simulink model "Noa_Nofusion_angle"  (R2020b)
settings: Solver=FixedStepDiscrete  StartTime=0.0  StopTime=Inf  FixedStep=0.01  RelTol=1e-3
PostLoadFcn:
  | if any(exist('dsrtsu_mdlpostloadfcn', 'file') ~= 0), dsrtsu_mdlpostloadfcn('Execute', bdroot); end
InitFcn:
  | , if any(exist('rtifpga_mdlclblib', 'file') ~= 0), rtifpga_mdlclblib('Init', bdroot); end,
  | , if any(exist('dsmpb_private', 'file') ~= 0), dsmpb_private('dsmpb_mdlclblib', 'Init', bdroot); end,
undefined symbols (not defined in the file): ACC_TimeGap_DecSetSwt, ACC_TimeGap_IncSetSwt, AccelPedalPosn, AccelPedalPosnVldty, AccelPedlPosnDiagc, AccPedalOverride, ACU_ShiftInProgress, ADAS_Posn_CurLane, AESSwtReq, ALC_SwtReq, BrkPedalSts, CC_ACC_CANCEL_OFFSwt, CC_ACC_CRUISE_OFFSwt, CC_ACC_DecSetSpd_SetSwt, CC_ACC_IncSetSpd_ResuSwt, CC_ACCSwtErr, CharSpd_ms, CSA_NODE, CURRENT_GEAR, CurrentGearValid, DiscIntNeverNeededParam, DrvDoorSts, DrvSBR, DrvTrqReqOvld, ECMACCInterface, ECMRespACC, ELKSwtReq, EngLimpHomeSts, EngSpd, EngState, EngState_PHEV, EngTrqMaxActSpd, EngTrqMinAct, EPS_DrvInpTrqVal_HighReslolution, EPS_FailSts, EPS_LKATorqOvrlDlvd, EPS_LKATorqOvrlDlvdVld, EPS_LKATrqOvlDlvdSts, EPS_SteerMod, EPS_TrqSnsrSts, EQ4_APPINFO, EQ4_LA_ELEM, EQ4_LA_HDR, EQ4_LAP_ELEM, EQ4_LAP_HDR, EQ4_LH_ELEM, EQ4_LH_HDR, EQ4_LRE_ELEM, EQ4_LRE_HDR, ESS_PedSwtReq, ESS_VehSwtReq, FFogLmpSts_F_Pbox, FLWheelDriveDirection, FLWheelSpd, FrntWiprSwtSts, FrntWshrSwtSts, FRWheelDriveDirection, FRWheelSpd, HazardLmpSwtSts, HCU_AccelPedalPosn_Diag ... (+151)
libraries: simulink x138, dsmpblib x33, canfdmsglib x10
(part 16 of 17)

== matlab function Noa_Nofusion_angle/CR_RSDS_Input/CR_R_Bus/CR ==
  data: RadarID input uint8 size=1; ID input uint8 size=6; Dx input single size=6; Dy input single size=6; Vx input single size=6; Vy input single size=6; Ax input single size=6; ObjIDK1 input uint8 size=6; P output uint8 size=6; ObjDx output single size=6; ObjDy output single size=6; ObjVx output single size=6; ObjVy output single size=6; ObjAx output single size=6; ObjMoveSts output uint8 size=6; ObjFusType output uint8 size=6; ObjID output uint8 size=6; ObjAgeK1 input uint8 size=6; ObjAge output uint8 size=6
function [P,ObjDx,ObjDy,ObjVx,ObjVy,ObjAx,ObjMoveSts,ObjFusType,ObjID,ObjAge] =...
    DataT(RadarID,ID,Dx,Dy,Vx,Vy,Ax,ObjIDK1,ObjAgeK1)

if RadarID==uint8(1)
    FusFac = 4;
elseif RadarID==uint8(2)
    FusFac = 8;
elseif RadarID==uint8(3)
    FusFac = 16;
else
    FusFac = 32;
end

ObjID = uint8(zeros(6,1));
ObjDx = single(zeros(6,1));
ObjDy = single(zeros(6,1));
ObjVx = single(zeros(6,1));
ObjVy = single(zeros(6,1));
ObjAx = single(zeros(6,1));
ObjAge = uint8(ones(6,1));
ObjMoveSts = uint8(2*ones(6,1));
ObjFusType = uint8(FusFac*ones(6,1));

T = uint8(zeros(6,1));
P = uint8(zeros(6,1));
Index01 = uint8(zeros(6,1));
Index02 = uint8(zeros(6,1));
M = uint8(0);
N = uint8(0);
w = uint8(0);

for i=uint8(1):uint8(6)
    for j=uint8(1):uint8(6)
        if ID(i)==ObjIDK1(j) && ID(i)>uint8(0)
            T(j) = i;
            P(i) = j;
        end
    end
end

for j=uint8(1):uint8(6)
    if T(j)==uint8(0)
        if ObjIDK1(j)==uint8(0)
            N = N + uint8(1);
            Index01(N) = j;
        else
            M = M + uint8(1);
            Index02(M) = j;
        end
    end
end

for i=uint8(1):uint8(6)
    if P(i)==uint8(0) && ID(i)>uint8(0)
        w = w + uint8(1);
        if w<=N
            P(i) = Index01(w);
        else
            P(i) = Index02(w - N);
        end
    elseif P(i)>uint8(0)
        ObjAge(P(i)) = min(ObjAgeK1(i) + uint8(1),uint8(255));
    end
    if P(i)>uint8(0)
       ObjID(P(i)) = ID(i);
       ObjDx(P(i)) = Dx(i);
       ObjDy(P(i)) = Dy(i);
       ObjVx(P(i)) = Vx(i);
       ObjVy(P(i)) = Vy(i);
       ObjAx(P(i)) = Ax(i);
    end
end
for i=uint8(1):uint8(6)
    if ObjID(i)==uint8(0)
        ObjAge(i) = uint8(0);
        ObjMoveSts(i) = uint8(0);
        ObjFusType(i) = uint8(0);
    end
end
end

== matlab function Noa_Nofusion_angle/TOS/Subsystem1/ACCOSM/HWA_Task100ms1/OTL1/MATLAB Function ==
  data: t input single; Valid output boolean; CutIn_b input boolean; ValidK1 input boolean
function Valid = fcn(t,CutIn_b,ValidK1)

if t<0.1
    Valid = false;
else
    if CutIn_b==false
       Valid = true; 
    else
       Valid = ValidK1;
    end
end

== matlab function Noa_Nofusion_angle/CR_RSDS_Input/MATLAB Function1 ==
  data: ObjNumber input uint8 size=1; ObjPrio output single size=24; ObjID input uint8 size=24; ObjDx input single size=24; ObjMatrix output single size=24
function [ObjPrio,ObjMatrix] = fcn(ObjNumber,ObjID,ObjDx)
%#codegen
ObjPrio = single(zeros(24,1));

for i=1:ObjNumber
    if ObjID(i)>0
        ObjPrio(i)=single(255) - abs(ObjDx(i));
    else
        ObjPrio(i)=single(0);
    end
end

ObjMatrix=ObjPrio;

t_h=1;
while 1
    t_h = t_h*3+1;
    if t_h>=ObjNumber
        break;
    end
end

%   t_h = 121;
while 1
    t_h = fix(t_h/3);
    for i=(t_h+1):ObjNumber
        j=i;
        t_zw=ObjMatrix(i);
        while (j>t_h)&&(t_zw<ObjMatrix(j-t_h))
            ObjMatrix(j)=ObjMatrix(j-t_h);
            j=j-t_h;
        end
        ObjMatrix(j)=t_zw;
    end
    if t_h==1
        break;
    end
end
end

== matlab function Noa_Nofusion_angle/CR_RSDS_Input/MATLAB Function2 ==
  data: Prio input single size=24; Matrix input single size=24; ID input uint8 size=24; ObjID output uint8 size=11; Dx input single size=24; Dy input single size=24; ObjDx output single size=11; Vx input single size=24; Vy input single size=24; Ax input single size=24; Age input uint8 size=24; MoveSts input uint8 size=24; ObjDy output single size=11; ObjVx output single size=11; ObjVy output single size=11; ObjAx output single size=11; ObjAge output uint8 size=11; ObjMoveSts output uint8 size=11; FusType input uint8 size=24; ObjFusType output uint8 size=11
function [ObjID,ObjDx,ObjDy,ObjVx,ObjVy,ObjAx,ObjAge,ObjMoveSts,ObjFusType] =...
    fcn(Prio,Matrix,ID,Dx,Dy,Vx,Vy,Ax,Age,MoveSts,FusType)
%#codegen
ObjPrioLimit = Matrix(24-11);
ObjID = uint8(zeros(11,1));
ObjDx = single(zeros(11,1));
ObjDy = single(zeros(11,1));
ObjVx = single(zeros(11,1));
ObjVy = single(zeros(11,1));
ObjAx = single(zeros(11,1));
ObjAge = uint8(zeros(11,1));
ObjMoveSts = uint8(zeros(11,1));
ObjFusType = uint8(zeros(11,1));
Num = uint8(0);

for i=1:24
  if ID(i)>0 && Prio(i)>ObjPrioLimit
      Num = Num + uint8(1);
      ObjID(Num) = uint8(i);
      ObjDx(Num) = Dx(i);
      ObjDy(Num) = Dy(i);
      ObjVx(Num) = Vx(i);
      ObjVy(Num) = Vy(i);
      ObjAx(Num) = Ax(i);
      ObjAge(Num) = Age(i);
      ObjMoveSts(Num) = MoveSts(i);
      ObjFusType(Num) = FusType(i);
  end
end

== matlab function Noa_Nofusion_angle/CR_RSDS_Input/RSDS_L_Bus/RSDS_L ==
  data: RadarID input uint8 size=1; ID input uint8 size=6; Dx input single size=6; Dy input single size=6; Vx input single size=6; Vy input single size=6; Ax input single size=6; ObjIDK1 input uint8 size=6; P output uint8 size=6; ObjDx output single size=6; ObjDy output single size=6; ObjVx output single size=6; ObjVy output single size=6; ObjAx output single size=6; ObjMoveSts output uint8 size=6; ObjFusType output uint8 size=6; ObjID output uint8 size=6; ObjAgeK1 input uint8 size=6; ObjAge output uint8 size=6
function [P,ObjDx,ObjDy,ObjVx,ObjVy,ObjAx,ObjMoveSts,ObjFusType,ObjID,ObjAge] =...
    DataT(RadarID,ID,Dx,Dy,Vx,Vy,Ax,ObjIDK1,ObjAgeK1)

if RadarID==uint8(1)
    FusFac = 4;
elseif RadarID==uint8(2)
    FusFac = 8;
elseif RadarID==uint8(3)
    FusFac = 16;
else
    FusFac = 32;
end

ObjID = uint8(zeros(6,1));
ObjDx = single(zeros(6,1));
ObjDy = single(zeros(6,1));
ObjVx = single(zeros(6,1));
ObjVy = single(zeros(6,1));
ObjAx = single(zeros(6,1));
ObjAge = uint8(ones(6,1));
ObjMoveSts = uint8(2*ones(6,1));
ObjFusType = uint8(FusFac*ones(6,1));

T = uint8(zeros(6,1));
P = uint8(zeros(6,1));
Index01 = uint8(zeros(6,1));
Index02 = uint8(zeros(6,1));
M = uint8(0);
N = uint8(0);
w = uint8(0);

for i=uint8(1):uint8(6)
    for j=uint8(1):uint8(6)
        if ID(i)==ObjIDK1(j) && ID(i)>uint8(0)
            T(j) = i;
            P(i) = j;
        end
    end
end

for j=uint8(1):uint8(6)
    if T(j)==uint8(0)
        if ObjIDK1(j)==uint8(0)
            N = N + uint8(1);
            Index01(N) = j;
        else
            M = M + uint8(1);
            Index02(M) = j;
        end
    end
end

for i=uint8(1):uint8(6)
    if P(i)==uint8(0) && ID(i)>uint8(0)
        w = w + uint8(1);
        if w<=N
            P(i) = Index01(w);
        else
            P(i) = Index02(w - N);
        end
    elseif P(i)>uint8(0)
        ObjAge(P(i)) = min(ObjAgeK1(i) + uint8(1),uint8(255));
    end
    if P(i)>uint8(0)
       ObjID(P(i)) = ID(i);
       ObjDx(P(i)) = Dx(i);
       ObjDy(P(i)) = Dy(i);
       ObjVx(P(i)) = Vx(i);
       ObjVy(P(i)) = Vy(i);
       ObjAx(P(i)) = Ax(i);
    end
end
for i=uint8(1):uint8(6)
    if ObjID(i)==uint8(0)
        ObjAge(i) = uint8(0);
        ObjMoveSts(i) = uint8(0);
        ObjFusType(i) = uint8(0);
    end
end
end

== matlab function Noa_Nofusion_angle/CR_RSDS_Input/RSDS_R_Bus/RSDS_R ==
  data: RadarID input uint8 size=1; ID input uint8 size=6; Dx input single size=6; Dy input single size=6; Vx input single size=6; Vy input single size=6; Ax input single size=6; ObjIDK1 input uint8 size=6; P output uint8 size=6; ObjDx output single size=6; ObjDy output single size=6; ObjVx output single size=6; ObjVy output single size=6; ObjAx output single size=6; ObjMoveSts output uint8 size=6; ObjFusType output uint8 size=6; ObjID output uint8 size=6; ObjAgeK1 input uint8 size=6; ObjAge output uint8 size=6
function [P,ObjDx,ObjDy,ObjVx,ObjVy,ObjAx,ObjMoveSts,ObjFusType,ObjID,ObjAge] =...
    DataT(RadarID,ID,Dx,Dy,Vx,Vy,Ax,ObjIDK1,ObjAgeK1)

if RadarID==uint8(1)
    FusFac = 4;
elseif RadarID==uint8(2)
    FusFac = 8;
elseif RadarID==uint8(3)
    FusFac = 16;
else
    FusFac = 32;
end

ObjID = uint8(zeros(6,1));
ObjDx = single(zeros(6,1));
ObjDy = single(zeros(6,1));
ObjVx = single(zeros(6,1));
ObjVy = single(zeros(6,1));
ObjAx = single(zeros(6,1));
ObjAge = uint8(ones(6,1));
ObjMoveSts = uint8(2*ones(6,1));
ObjFusType = uint8(FusFac*ones(6,1));

T = uint8(zeros(6,1));
P = uint8(zeros(6,1));
Index01 = uint8(zeros(6,1));
Index02 = uint8(zeros(6,1));
M = uint8(0);
N = uint8(0);
w = uint8(0);

for i=uint8(1):uint8(6)
    for j=uint8(1):uint8(6)
        if ID(i)==ObjIDK1(j) && ID(i)>uint8(0)
            T(j) = i;
            P(i) = j;
        end
    end
end

for j=uint8(1):uint8(6)
    if T(j)==uint8(0)
        if ObjIDK1(j)==uint8(0)
            N = N + uint8(1);
            Index01(N) = j;
        else
            M = M + uint8(1);
            Index02(M) = j;
        end
    end
end

for i=uint8(1):uint8(6)
    if P(i)==uint8(0) && ID(i)>uint8(0)
        w = w + uint8(1);
        if w<=N
            P(i) = Index01(w);
        else
            P(i) = Index02(w - N);
        end
    elseif P(i)>uint8(0)
        ObjAge(P(i)) = min(ObjAgeK1(i) + uint8(1),uint8(255));
    end
    if P(i)>uint8(0)
       ObjID(P(i)) = ID(i);
       ObjDx(P(i)) = Dx(i);
       ObjDy(P(i)) = Dy(i);
       ObjVx(P(i)) = Vx(i);
       ObjVy(P(i)) = Vy(i);
       ObjAx(P(i)) = Ax(i);
    end
end
for i=uint8(1):uint8(6)
    if ObjID(i)==uint8(0)
        ObjAge(i) = uint8(0);
        ObjMoveSts(i) = uint8(0);
        ObjFusType(i) = uint8(0);
    end
end
end

== matlab function Noa_Nofusion_angle/TOS/Subsystem1/ACCOSM/HWA_Task100ms1/OTL1/P0TrajHistCalc01 ==
  data: P0Dyc output; vRef input; tCycle input single; tSameHandle input single; CutIn input; P0Dx input single; P0Dy input single; P0TrajHistNum output uint8; EgoDDeltaX input single; EgoDDeltaY input single; EgoCosOfPsi input single; EgoSinOfPsi input single; TarLineValid input; TarLineA2 input; TarLineA1 input; TarLineA0 input; P0TrajHistDxv output single; P0TrajHistDyv output single; P0TrajHistNumK1 input uint8; P0TrajHistDxvK1 input single; P0TrajHistDyvK1 input single
function [P0Dyc,P0TrajHistNum,P0TrajHistDxv,P0TrajHistDyv]...
    = fcn(vRef, tCycle,tSameHandle,CutIn, P0Dx,P0Dy,EgoDDeltaX,EgoDDeltaY,EgoCosOfPsi,EgoSinOfPsi,...
    TarLineValid,TarLineA2,TarLineA1,TarLineA0,...
    P0TrajHistNumK1,P0TrajHistDxvK1,P0TrajHistDyvK1)
%#codegen
P0TrajHistNum = P0TrajHistNumK1;
P0TrajHistDxv = P0TrajHistDxvK1;
P0TrajHistDyv = P0TrajHistDyvK1;

if TarLineValid
    temp1 = TarLineA2*P0Dx*P0Dx + TarLineA1*P0Dx + TarLineA0;
    P0Dyc = P0Dy - temp1;
else
    P0Dyc = single(255);
end
                
if tSameHandle==0
    P0TrajHistNum = uint8(0);
    P0TrajHistDxv = single(zeros(24,1));
    P0TrajHistDyv = single(zeros(24,1));
else
    if tSameHandle==tCycle
        if (CutIn&&abs(P0Dyc)>0.5) || (abs(P0Dyc)>0.8)||(vRef>8)
            P0TrajHistDxv(1) = P0Dx;
            P0TrajHistDyv(1) = P0Dy;
            P0TrajHistNum = uint8(1);
        else
            P0TrajHistDxv(1) = P0Dx;
            P0TrajHistDyv(1) = P0Dy;
            P0TrajHistNum = uint8(1);
            
            if TarLineValid
                P0TrajHistDxv(2) = 0.6*P0Dx;
                temp2 = 0.36*TarLineA2*P0Dx*P0Dx + 0.6*TarLineA1*P0Dx + TarLineA0;
                P0TrajHistDyv(2) = P0Dyc + temp2;
                
                P0TrajHistDxv(3) = 0.3*P0Dx;
                temp3 = 0.09*TarLineA2*P0Dx*P0Dx + 0.3*TarLineA1*P0Dx + TarLineA0;
                P0TrajHistDyv(3) = P0Dyc + temp3;
                
                P0TrajHistDxv(4) = single(-1);
                temp4 = TarLineA2 - TarLineA1 + TarLineA0;
                P0TrajHistDyv(4) = P0Dyc + temp4;
                
                P0TrajHistNum = uint8(4);
            end
        end
    else
        Temp1 = P0TrajHistDxv(1) - EgoDDeltaX - P0Dx;
        Temp2 = P0TrajHistDyv(1) - EgoDDeltaY - P0Dy;
        dDeltaS = Temp1*Temp1 + Temp2*Temp2;
        
        t_d = interpolate(single(8),single(0.5),single(22),single(2.5),single(P0TrajHistNum));
        t_d = t_d*t_d;
        t_AddPosition = (dDeltaS>t_d);
        
        for iBuf=1:P0TrajHistNum
            dX = P0TrajHistDxv(iBuf)-EgoDDeltaX;
            dY = P0TrajHistDyv(iBuf)-EgoDDeltaY;
            P0TrajHistDxv(iBuf) = dX*EgoCosOfPsi + dY*EgoSinOfPsi;
            P0TrajHistDyv(iBuf) = -dX*EgoSinOfPsi + dY*EgoCosOfPsi;
            if (P0TrajHistDxv(iBuf)<-5)||(abs(P0TrajHistDyv(iBuf))>50)
                P0TrajHistNum = max(P0TrajHistNum - uint8(1),uint8(0));
            end
        end
        
        if t_AddPosition==true
            
            P0TrajHistNum = min(P0TrajHistNum + uint8(1),uint8(24));
            for iBuf= P0TrajHistNum:(-1):2
                P0TrajHistDxv(iBuf) = P0TrajHistDxv(iBuf-uint8(1));
                P0TrajHistDyv(iBuf) = P0TrajHistDyv(iBuf-uint8(1));
            end
            P0TrajHistDxv(1) = P0Dx;
            P0TrajHistDyv(1) = P0Dy;
        end
    end
end
end

function out = interpolate(x1,z1,x2,z2,Raw)
if Raw<=x1
    out = z1;
else
    if Raw>=x2
        out = z2;
    else
        out = z1 + (Raw-x1)*(z2-z1)/(x2-x1);
    end
end
end

== matlab function Noa_Nofusion_angle/SimBCM/BCMsim ==
  data: SimLeLmp input; CSASim_LampReq output; SimRiLmp input; Model_IDC_L2_LampReq input
function CSASim_LampReq = fcn(SimLeLmp, SimRiLmp, Model_IDC_L2_LampReq)
CSASim_LampReq=Model_IDC_L2_LampReq;
if SimRiLmp
    CSASim_LampReq=uint8(2);
end
if SimLeLmp
    CSASim_LampReq=uint8(1);
end

== matlab function Noa_Nofusion_angle/TOS/Subsystem1/ACCOSM/HWA_Task100ms1/OTL1/P0TrajHistCalc1 ==
  data: P0TrajHistNum output uint8; P0TrajHistNum1 input uint8; P0TrajHistDxv1 input single; P0TrajHistDxv output single; P0TrajHistDyv1 input single; P0TrajHistDyv output single; LineValid output boolean; a output single; b output single; c output single; d output single; dxMin output single; dxMax output single
function [P0TrajHistNum,P0TrajHistDxv,P0TrajHistDyv,LineValid,a,b,c,d,dxMin,dxMax] = P0TrajHistMixCalc(...
    P0TrajHistNum1,P0TrajHistDxv1,P0TrajHistDyv1)

P0TrajHistDxv = single(zeros(48,1));
P0TrajHistDyv = single(zeros(48,1));
P0TrajHistNum = uint8(0);

if (P0TrajHistNum1>0)
    P0TrajHistDxv(1:P0TrajHistNum1) = P0TrajHistDxv1(1:P0TrajHistNum1);
    P0TrajHistDyv(1:P0TrajHistNum1) = P0TrajHistDyv1(1:P0TrajHistNum1);
    P0TrajHistNum = P0TrajHistNum1;
end

if P0TrajHistNum>=4
    dxMin = P0TrajHistDxv(P0TrajHistNum);
    dxMax = P0TrajHistDxv(1) + 6;
%     q2 = max(ceil(P0TrajHistNum/2),2);
%     q3 = max(ceil(P0TrajHistNum*3/4),3);
%     q4 = P0TrajHistNum;
%     MaX = [P0TrajHistDxv(1);P0TrajHistDxv(q2);P0TrajHistDxv(q3);P0TrajHistDxv(q4)];
%     MaY = [P0TrajHistDyv(1);P0TrajHistDyv(q2);P0TrajHistDyv(q3);P0TrajHistDyv(q4)];
%     [~,b,c,d] = pl(MaX,MaY);
    P = polyfit(P0TrajHistDxv(1:P0TrajHistNum),P0TrajHistDyv(1:P0TrajHistNum),2);
    b = P(1);
    c = P(2);
    d = P(3);

    a = single(0);
   LineValid = true;
   if dxMin>0.5
      LineValid = false; 
   end
else
   dxMin = single(0); 
   dxMax = single(0); 
   a = single(0);
   b = single(0);
   c = single(0);
   d = single(0);
   LineValid = false;
end

== stateflow chart Noa_Nofusion_angle/SimBCM/CSALampCtrlSim/Chart1 ==
  state OFF
    en:
    SwtSts=false;
  state Hold
    en:
    SwtSts=true;
  state LeCloseReady
  (default) -> OFF
  LeCloseReady -> OFF : [SteerWheelAng<P_LmpCloseAngClose...
      | ||OFF]
  Hold -> OFF [order 2] : [OFF]
  OFF -> Hold : [ON]
  Hold -> LeCloseReady [order 1] : [SteerWheelAng>P_LmpCloseAngReady]
  data: SwtSts output; OFF input; ON input; SteerWheelAng input; P_LmpCloseAngClose input; P_LmpCloseAngReady input

== matlab function Noa_Nofusion_angle/Subsystem4/LHLine ==
  data: LH_Count input; LH1A0 input single size=1; LH1A1 input single size=1; LH1A2 input single size=1; LH1A3 input single size=1; LH1RaMin input single size=1; LH1RaMax input single size=1; LH1Conf output uint8 size=1; LH1Avail input uint8 size=1; LH1LineType input uint8 size=1; LH1DLType input uint8 size=1; LH1SideType input uint8 size=1; LH1Wid input single size=1; LH1Crossing input; LH1Confidence input; LH2A0 input single size=1; LH2A1 input single size=1; LH2A2 input single size=1; LH2A3 input single size=1; LH2RaMin input single size=1; LH2RaMax input single size=1; LH2Avail input uint8 size=1; LH2LineType input uint8 size=1; LH2DLType input uint8 size=1; LH2SideType input uint8 size=1; LH2Wid input single size=1; LH1C0 output single size=1; LH1C1 output single size=1; LH1C2 output single size=1; LH1C3 output single size=1; LH1DxMin output single size=1; LH1DxMax output single size=1; LH1Type output uint8 size=1; LH1DLM output uint8 size=1; LH1Width output single size=1; LH1Reliable output; LeftLaneChange output uint8 size=1; LH2Conf output uint8 size=1; LH2C0 output single size=1; LH2C1 output single size=1; LH2C2 output single size=1; LH2C3 output single size=1; LH2DxMin output single size=1; LH2DxMax output single size=1; LH2Type output uint8 size=1; LH2DLM output uint8 size=1; LH2Width output single size=1; LH2Reliable output; RightLaneChange output uint8 size=1; LH2Crossing input; LH2Confidence input
function [LH1Conf,LH1C0,LH1C1,LH1C2,LH1C3,LH1DxMin,LH1DxMax,LH1Type,LH1DLM,LH1Width,LH1Reliable,LeftLaneChange,...
    LH2Conf,LH2C0,LH2C1,LH2C2,LH2C3,LH2DxMin,LH2DxMax,LH2Type,LH2DLM,LH2Width,LH2Reliable,RightLaneChange]...
    = LH(LH_Count,LH1A0,LH1A1,LH1A2,LH1A3,LH1RaMin,LH1RaMax,LH1Avail,LH1LineType,LH1DLType,LH1SideType,LH1Wid,LH1Crossing,LH1Confidence,...
    LH2A0,LH2A1,LH2A2,LH2A3,LH2RaMin,LH2RaMax,LH2Avail,LH2LineType,LH2DLType,LH2SideType,LH2Wid,LH2Crossing,LH2Confidence)

LH1Conf = uint8(0);
LH1C0 = single(0);
LH1C1 = single(0);
LH1C2 = single(0);
LH1C3 = single(0);
LH1DxMin = single(0);
LH1DxMax = single(0);
LH1Type = uint8(0);
LH1DLM = uint8(0);
LH1Width = single(0);
LH1Reliable = single(0);
LeftLaneChange = uint8(0);

LH2Conf = uint8(0);
LH2C0 = single(0);
LH2C1 = single(0);
LH2C2 = single(0);
LH2C3 = single(0);
LH2DxMin = single(0);
LH2DxMax = single(0);
LH2Type = uint8(0);
LH2DLM = uint8(0);
LH2Width = single(0);
LH2Reliable = single(0);
RightLaneChange = uint8(0);


%%
if LH_Count >= 1
    if LH1SideType==1
        LH1Conf = LH1Avail;
        LH1C0 = LH1A0;
        LH1C1 = LH1A1;
        LH1C2 = LH1A2;
        LH1C3 = LH1A3;
        LH1DxMin = LH1RaMin;
        LH1DxMax = LH1RaMax;
        LH1Type = LH1LineType;
        LH1DLM = LH1DLType;
        LH1Width = LH1Wid;
        LH1Reliable = LH1Confidence;
        LeftLaneChange = LH1Crossing;
    elseif LH1SideType==2
        LH2Conf = LH1Avail;
        LH2C0 = LH1A0;
        LH2C1 = LH1A1;
        LH2C2 = LH1A2;
        LH2C3 = LH1A3;
        LH2DxMin = LH1RaMin;
        LH2DxMax = LH1RaMax;
        LH2Type = LH1LineType;
        LH2DLM = LH1DLType;
        LH2Width = LH1Wid;
        LH2Reliable = LH1Confidence;
        RightLaneChange = LH1Crossing;
    end
    if LH_Count >= 2
        if LH2SideType==1
            LH1Conf = LH2Avail;
            LH1C0 = LH2A0;
            LH1C1 = LH2A1;
            LH1C2 = LH2A2;
            LH1C3 = LH2A3;
            LH1DxMin = LH2RaMin;
            LH1DxMax = LH2RaMax;
            LH1Type = LH2LineType;
            LH1DLM = LH2DLType;
            LH1Width = LH2Wid;
            LH1Reliable = LH2Confidence;
            LeftLaneChange = LH2Crossing;
        elseif LH2SideType==2
            LH2Conf = LH2Avail;
            LH2C0 = LH2A0;
            LH2C1 = LH2A1;
            LH2C2 = LH2A2;
            LH2C3 = LH2A3;
            LH2DxMin = LH2RaMin;
            LH2DxMax = LH2RaMax;
            LH2Type = LH2LineType;
            LH2DLM = LH2DLType;
            LH2Width = LH2Wid;
            LH2Reliable = LH2Confidence;
            RightLaneChange = LH2Crossing;
        end
    end
end

== matlab function Noa_Nofusion_angle/Subsystem4/MATLAB Function5 ==
  data: IFV2RearAxis input single size=1; a0 output single size=1; a1 output single size=1; a2 output single size=1; a3 output single size=1; IFV2CenterAxis input single size=1; A0 input single size=1; A1 input single size=1; A2 input single size=1; A3 input single size=1; Range_min input single size=1; Rmin output single size=1; Range_max input single size=1; Rmax output single size=1
function [a0,a1,a2,a3,Rmin,Rmax] = ...
    fcn(IFV2RearAxis,IFV2CenterAxis,A0,A1,A2,A3,Range_min,Range_max)

Rmin = Range_min + IFV2RearAxis;
Rmax = Range_max + IFV2RearAxis;

if Range_max>0
   xi = [10;20;40;80];
   yi = -A3*xi.^3 - A2*xi.^2 - A1*xi - A0 + IFV2CenterAxis;
   xi = xi + IFV2RearAxis;
   [a3,a2,a1,a0] = pl(xi,yi);
else
    a3 = single(0);
    a2 = single(0);
    a1 = single(0);
    a0 = single(0);
end

== matlab function Noa_Nofusion_angle/Subsystem4/MATLAB Function6 ==
  data: IFV2RearAxis input single size=1; a0 output single size=1; a1 output single size=1; a2 output single size=1; a3 output single size=1; IFV2CenterAxis input single size=1; A0 input single size=1; A1 input single size=1; A2 input single size=1; A3 input single size=1; Range_min input single size=1; Rmin output single size=1; Range_max input single size=1; Rmax output single size=1
function [a0,a1,a2,a3,Rmin,Rmax] = ...
    fcn(IFV2RearAxis,IFV2CenterAxis,A0,A1,A2,A3,Range_min,Range_max)

Rmin = Range_min + IFV2RearAxis;
Rmax = Range_max + IFV2RearAxis;

if Range_max>0
   xi = [10;20;40;80];
   yi = -A3*xi.^3 - A2*xi.^2 - A1*xi - A0 + IFV2CenterAxis;
   xi = xi + IFV2RearAxis;
   [a3,a2,a1,a0] = pl(xi,yi);
else
    a3 = single(0);
    a2 = single(0);
    a1 = single(0);
    a0 = single(0);
end

== matlab function Noa_Nofusion_angle/Subsystem4/Simulink Function/MATLAB Function3 ==
  data: IFV2RearAxis input single size=1; a0 output single size=1; a1 output single size=1; a2 output single size=1; a3 output single size=1; IFV2CenterAxis input single size=1; A0 input single size=1; A1 input single size=1; A2 input single size=1; A3 input single size=1; Range_min input single size=1; Rmin output single size=1; Range_max input single size=1; Rmax output single size=1
function [a0,a1,a2,a3,Rmin,Rmax] = ...
    fcn(IFV2RearAxis,IFV2CenterAxis,A0,A1,A2,A3,Range_min,Range_max)

Rmin = Range_min + IFV2RearAxis;
Rmax = Range_max + IFV2RearAxis;

if Range_max>0
   xi = [10;20;40;80];
   yi = -A3*xi.^3 - A2*xi.^2 - A1*xi - A0 + IFV2CenterAxis;
   xi = xi + IFV2RearAxis;
   [a3,a2,a1,a0] = pl(xi,yi);
else
    a3 = single(0);
    a2 = single(0);
    a1 = single(0);
    a0 = single(0);
end

== matlab function Noa_Nofusion_angle/Subsystem5/LHLine ==
  data: LH_Count input; LH1A0 input single size=1; LH1A1 input single size=1; LH1A2 input single size=1; LH1A3 input single size=1; LH1RaMin input single size=1; LH1RaMax input single size=1; LH1Conf output uint8 size=1; LH1Avail input uint8 size=1; LH1LineType input uint8 size=1; LH1DLType input uint8 size=1; LH1SideType input uint8 size=1; LH1Wid input single size=1; LH1Crossing input; LH1Confidence input; LH2A0 input single size=1; LH2A1 input single size=1; LH2A2 input single size=1; LH2A3 input single size=1; LH2RaMin input single size=1; LH2RaMax input single size=1; LH2Avail input uint8 size=1; LH2LineType input uint8 size=1; LH2DLType input uint8 size=1; LH2SideType input uint8 size=1; LH2Wid input single size=1; LH1C0 output single size=1; LH1C1 output single size=1; LH1C2 output single size=1; LH1C3 output single size=1; LH1DxMin output single size=1; LH1DxMax output single size=1; LH1Type output uint8 size=1; LH1DLM output uint8 size=1; LH1Width output single size=1; LH1Reliable output; LeftLaneChange output uint8 size=1; LH2Conf output uint8 size=1; LH2C0 output single size=1; LH2C1 output single size=1; LH2C2 output single size=1; LH2C3 output single size=1; LH2DxMin output single size=1; LH2DxMax output single size=1; LH2Type output uint8 size=1; LH2DLM output uint8 size=1; LH2Width output single size=1; LH2Reliable output; RightLaneChange output uint8 size=1; LH2Crossing input; LH2Confidence input
function [LH1Conf,LH1C0,LH1C1,LH1C2,LH1C3,LH1DxMin,LH1DxMax,LH1Type,LH1DLM,LH1Width,LH1Reliable,LeftLaneChange,...
    LH2Conf,LH2C0,LH2C1,LH2C2,LH2C3,LH2DxMin,LH2DxMax,LH2Type,LH2DLM,LH2Width,LH2Reliable,RightLaneChange]...
    = LH(LH_Count,LH1A0,LH1A1,LH1A2,LH1A3,LH1RaMin,LH1RaMax,LH1Avail,LH1LineType,LH1DLType,LH1SideType,LH1Wid,LH1Crossing,LH1Confidence,...
    LH2A0,LH2A1,LH2A2,LH2A3,LH2RaMin,LH2RaMax,LH2Avail,LH2LineType,LH2DLType,LH2SideType,LH2Wid,LH2Crossing,LH2Confidence)

LH1Conf = uint8(0);
LH1C0 = single(0);
LH1C1 = single(0);
LH1C2 = single(0);
LH1C3 = single(0);
LH1DxMin = single(0);
LH1DxMax = single(0);
LH1Type = uint8(0);
LH1DLM = uint8(0);
LH1Width = single(0);
LH1Reliable = single(0);
LeftLaneChange = uint8(0);

LH2Conf = uint8(0);
LH2C0 = single(0);
LH2C1 = single(0);
LH2C2 = single(0);
LH2C3 = single(0);
LH2DxMin = single(0);
LH2DxMax = single(0);
LH2Type = uint8(0);
LH2DLM = uint8(0);
LH2Width = single(0);
LH2Reliable = single(0);
RightLaneChange = uint8(0);


%%
if LH_Count >= 1
    if LH1SideType==1
        LH1Conf = LH1Avail;
        LH1C0 = LH1A0;
        LH1C1 = LH1A1;
        LH1C2 = LH1A2;
        LH1C3 = LH1A3;
        LH1DxMin = LH1RaMin;
        LH1DxMax = LH1RaMax;
        LH1Type = LH1LineType;
        LH1DLM = LH1DLType;
        LH1Width = LH1Wid;
        LH1Reliable = LH1Confidence;
        LeftLaneChange = LH1Crossing;
    elseif LH1SideType==2
        LH2Conf = LH1Avail;
        LH2C0 = LH1A0;
        LH2C1 = LH1A1;
        LH2C2 = LH1A2;
        LH2C3 = LH1A3;
        LH2DxMin = LH1RaMin;
        LH2DxMax = LH1RaMax;
        LH2Type = LH1LineType;
        LH2DLM = LH1DLType;
        LH2Width = LH1Wid;
        LH2Reliable = LH1Confidence;
        RightLaneChange = LH1Crossing;
    end
    if LH_Count >= 2
        if LH2SideType==1
            LH1Conf = LH2Avail;
            LH1C0 = LH2A0;
            LH1C1 = LH2A1;
            LH1C2 = LH2A2;
            LH1C3 = LH2A3;
            LH1DxMin = LH2RaMin;
            LH1DxMax = LH2RaMax;
            LH1Type = LH2LineType;
            LH1DLM = LH2DLType;
            LH1Width = LH2Wid;
            LH1Reliable = LH2Confidence;
            LeftLaneChange = LH2Crossing;
        elseif LH2SideType==2
            LH2Conf = LH2Avail;
            LH2C0 = LH2A0;
            LH2C1 = LH2A1;
            LH2C2 = LH2A2;
            LH2C3 = LH2A3;
            LH2DxMin = LH2RaMin;
            LH2DxMax = LH2RaMax;
            LH2Type = LH2LineType;
            LH2DLM = LH2DLType;
            LH2Width = LH2Wid;
            LH2Reliable = LH2Confidence;
            RightLaneChange = LH2Crossing;
        end
    end
end

== matlab function Noa_Nofusion_angle/Subsystem5/MATLAB Function5 ==
  data: IFV2RearAxis input single size=1; a0 output single size=1; a1 output single size=1; a2 output single size=1; a3 output single size=1; IFV2CenterAxis input single size=1; A0 input single size=1; A1 input single size=1; A2 input single size=1; A3 input single size=1; Range_min input single size=1; Rmin output single size=1; Range_max input single size=1; Rmax output single size=1
function [a0,a1,a2,a3,Rmin,Rmax] = ...
    fcn(IFV2RearAxis,IFV2CenterAxis,A0,A1,A2,A3,Range_min,Range_max)

Rmin = Range_min + IFV2RearAxis;
Rmax = Range_max + IFV2RearAxis;

if Range_max>0
   xi = [10;20;40;80];
   yi = -A3*xi.^3 - A2*xi.^2 - A1*xi - A0 + IFV2CenterAxis;
   xi = xi + IFV2RearAxis;
   [a3,a2,a1,a0] = pl(xi,yi);
else
    a3 = single(0);
    a2 = single(0);
    a1 = single(0);
    a0 = single(0);
end

== matlab function Noa_Nofusion_angle/Subsystem5/MATLAB Function6 ==
  data: IFV2RearAxis input single size=1; a0 output single size=1; a1 output single size=1; a2 output single size=1; a3 output single size=1; IFV2CenterAxis input single size=1; A0 input single size=1; A1 input single size=1; A2 input single size=1; A3 input single size=1; Range_min input single size=1; Rmin output single size=1; Range_max input single size=1; Rmax output single size=1
function [a0,a1,a2,a3,Rmin,Rmax] = ...
    fcn(IFV2RearAxis,IFV2CenterAxis,A0,A1,A2,A3,Range_min,Range_max)

Rmin = Range_min + IFV2RearAxis;
Rmax = Range_max + IFV2RearAxis;

if Range_max>0
   xi = [10;20;40;80];
   yi = -A3*xi.^3 - A2*xi.^2 - A1*xi - A0 + IFV2CenterAxis;
   xi = xi + IFV2RearAxis;
   [a3,a2,a1,a0] = pl(xi,yi);
else
    a3 = single(0);
    a2 = single(0);
    a1 = single(0);
    a0 = single(0);
end

== stateflow chart Noa_Nofusion_angle/SimBCM/CSALampCtrlSim/Chart2 ==
  state OFF
    en:
    SwtSts=false;
  state Hold
    en:
    SwtSts=true;
  state LeCloseReady
  (default) -> OFF
  LeCloseReady -> OFF : [abs(SteerWheelAng)>-P_LmpCloseAngClose...
      | ||OFF]
  Hold -> OFF [order 2] : [OFF]
  OFF -> Hold : [ON]
  Hold -> LeCloseReady [order 1] : [SteerWheelAng<-P_LmpCloseAngReady]
  data: SwtSts output; OFF input; ON input; SteerWheelAng input; P_LmpCloseAngClose input; P_LmpCloseAngReady input

== matlab function Noa_Nofusion_angle/Subsystem4/LALine ==
  data: LA_Count input; L1Conf output uint8 size=1; L1C0 output single size=1; L1C1 output single size=1; L1C2 output single size=1; L1C3 output single size=1; L1DxMin output single size=1; L1DxMax output single size=1; L1A0 input single size=1; L1A1 input single size=1; L1A2 input single size=1; L1A3 input single size=1; L1RaMin input single size=1; L1RaMax input single size=1; L1Avail input uint8 size=1; L1LineType input uint8 size=1; L1DLType input uint8 size=1; L1SideType input uint8 size=1; L1Wid input single size=1; L1Confidence input; L2A0 input single size=1; L2A1 input single size=1; L2A2 input single size=1; L2A3 input single size=1; L2RaMin input single size=1; L2RaMax input single size=1; L2Avail input uint8 size=1; L2LineType input uint8 size=1; L2DLType input uint8 size=1; L2SideType input uint8 size=1; L2Wid input single size=1; L2Confidence input; L3A0 input single size=1; L3A1 input single size=1; L3A2 input single size=1; L3A3 input single size=1; L3RaMin input single size=1; L3RaMax input single size=1; L3Avail input uint8 size=1; L3LineType input uint8 size=1; L3DLType input uint8 size=1; L3SideType input uint8 size=1; L3Wid input single size=1; L3Confidence input; L4A0 input single size=1; L4A1 input single size=1; L4A2 input single size=1; L4A3 input single size=1; L4RaMin input single size=1; L4RaMax input single size=1; L4Avail input uint8 size=1; L4LineType input uint8 size=1; L4DLType input uint8 size=1; L4SideType input uint8 size=1; L4Wid input single size=1; L1Type output uint8 size=1; L1DLM output uint8 size=1; L1Width output single size=1; L1Reliable output; L2Conf output uint8 size=1; L2C0 output single size=1; L2C1 output single size=1; L2C2 output single size=1; L2C3 output single size=1; L2DxMin output single size=1; L2DxMax output single size=1; L2Type output uint8 size=1; L2DLM output uint8 size=1; L2Width output single size=1; L2Reliable output; L3Conf output uint8 size=1; L3C0 output single size=1; L3C1 output single size=1; L3C2 output single size=1; L3C3 output single size=1; L3DxMin output single size=1; L3DxMax output single size=1; L3Type output uint8 size=1; L3DLM output uint8 size=1; L3Width output single size=1; L3Reliable output; L4Conf output uint8 size=1; L4C0 output single size=1; L4C1 output single size=1; L4C2 output single size=1; L4C3 output single size=1; L4DxMin output single size=1; L4DxMax output single size=1; L4Type output uint8 size=1; L4DLM output uint8 size=1; L4Width output single size=1; L4Confidence input; L4Reliable output
function [L1Conf,L1C0,L1C1,L1C2,L1C3,L1DxMin,L1DxMax,L1Type,L1DLM,L1Width,L1Reliable,...
    L2Conf,L2C0,L2C1,L2C2,L2C3,L2DxMin,L2DxMax,L2Type,L2DLM,L2Width,L2Reliable,...
    L3Conf,L3C0,L3C1,L3C2,L3C3,L3DxMin,L3DxMax,L3Type,L3DLM,L3Width,L3Reliable,...
    L4Conf,L4C0,L4C1,L4C2,L4C3,L4DxMin,L4DxMax,L4Type,L4DLM,L4Width,L4Reliable]...
    = LA(LA_Count,L1A0,L1A1,L1A2,L1A3,L1RaMin,L1RaMax,L1Avail,L1LineType,L1DLType,L1SideType,L1Wid,L1Confidence,...
    L2A0,L2A1,L2A2,L2A3,L2RaMin,L2RaMax,L2Avail,L2LineType,L2DLType,L2SideType,L2Wid,L2Confidence,...
    L3A0,L3A1,L3A2,L3A3,L3RaMin,L3RaMax,L3Avail,L3LineType,L3DLType,L3SideType,L3Wid,L3Confidence,...
    L4A0,L4A1,L4A2,L4A3,L4RaMin,L4RaMax,L4Avail,L4LineType,L4DLType,L4SideType,L4Wid,L4Confidence)

L1Conf = uint8(0);
L1C0 = single(0);
L1C1 = single(0);
L1C2 = single(0);
L1C3 = single(0);
L1DxMin = single(0);
L1DxMax = single(0);
L1Type = uint8(0);
L1DLM = uint8(0);
L1Width = single(0);
L1Reliable = single(0);

L2Conf = uint8(0);
L2C0 = single(0);
L2C1 = single(0);
L2C2 = single(0);
L2C3 = single(0);
L2DxMin = single(0);
L2DxMax = single(0);
L2Type = uint8(0);
L2DLM = uint8(0);
L2Width = single(0);
L2Reliable = single(0);

L3Conf = uint8(0);
L3C0 = single(0);
L3C1 = single(0);
L3C2 = single(0);
L3C3 = single(0);
L3DxMin = single(0);
L3DxMax = single(0);
L3Type = uint8(0);
L3DLM = uint8(0);
L3Width = single(0);
L3Reliable = single(0);

L4Conf = uint8(0);
L4C0 = single(0);
L4C1 = single(0);
L4C2 = single(0);
L4C3 = single(0);
L4DxMin = single(0);
L4DxMax = single(0);
L4Type = uint8(0);
L4DLM = uint8(0);
L4Width = single(0);
L4Reliable = single(0);
%%  临车道车道线预处理
if LA_Count >= 1                                     %临车道车道线数量
    if L1SideType==1                                 %左左车道线
        L1Conf = L1Avail;
        L1C0 = L1A0;
        L1C1 = L1A1;
        L1C2 = L1A2;
        L1C3 = L1A3;
        L1DxMin = L1RaMin;
        L1DxMax = L1RaMax;
        L1Type = L1LineType;
        L1DLM = L1DLType;
        L1Width = L1Wid;
        L1Reliable = L1Confidence;
    elseif L1SideType==2                             %左车道右侧车道线
        L2Conf = L1Avail;
        L2C0 = L1A0;
        L2C1 = L1A1;
        L2C2 = L1A2;
        L2C3 = L1A3;
        L2DxMin = L1RaMin;
        L2DxMax = L1RaMax;
        L2Type = L1LineType;
        L2DLM = L1DLType;
        L2Width = L1Wid;
        L2Reliable = L1Confidence;
    elseif L1SideType==3                             %右车道左侧车道线
        L3Conf = L1Avail;
        L3C0 = L1A0;
        L3C1 = L1A1;
        L3C2 = L1A2;
        L3C3 = L1A3;
        L3DxMin = L1RaMin;
        L3DxMax = L1RaMax;
        L3Type = L1LineType;
        L3DLM = L1DLType;
        L3Width = L1Wid;
        L3Reliable = L1Confidence;
    elseif L1SideType==4                             %右右车道线
        L4Conf = L1Avail;
        L4C0 = L1A0;
        L4C1 = L1A1;
        L4C2 = L1A2;
        L4C3 = L1A3;
        L4DxMin = L1RaMin;
        L4DxMax = L1RaMax;
        L4Type = L1LineType;
        L4DLM = L1DLType;
        L4Width = L1Wid;
        L4Reliable = L1Confidence;
    end
    if LA_Count >= 2
        if L2SideType==1
            L1Conf = L2Avail;
            L1C0 = L2A0;
            L1C1 = L2A1;
            L1C2 = L2A2;
            L1C3 = L2A3;
            L1DxMin = L2RaMin;
            L1DxMax = L2RaMax;
            L1Type = L2LineType;
            L1DLM = L2DLType;
            L1Width = L2Wid;
            L1Reliable = L2Confidence;
        elseif L2SideType==2
            L2Conf = L2Avail;
            L2C0 = L2A0;
            L2C1 = L2A1;
            L2C2 = L2A2;
            L2C3 = L2A3;
            L2DxMin = L2RaMin;
            L2DxMax = L2RaMax;
            L2Type = L2LineType;
            L2DLM = L2DLType;
            L2Width = L2Wid;
            L2Reliable = L2Confidence;
        elseif L2SideType==3
            L3Conf = L2Avail;
            L3C0 = L2A0;
            L3C1 = L2A1;
            L3C2 = L2A2;
            L3C3 = L2A3;
            L3DxMin = L2RaMin;
            L3DxMax = L2RaMax;
            L3Type = L2LineType;
            L3DLM = L2DLType;
            L3Width = L2Wid;
            L3Reliable = L2Confidence;
        elseif L2SideType==4
            L4Conf = L2Avail;
            L4C0 = L2A0;
            L4C1 = L2A1;
            L4C2 = L2A2;
            L4C3 = L2A3;
            L4DxMin = L2RaMin;
            L4DxMax = L2RaMax;
            L4Type = L2LineType;
            L4DLM = L2DLType;
            L4Width = L2Wid;
            L4Reliable = L2Confidence;
        end
        if LA_Count >= 3
            if L3SideType==1
                L1Conf = L3Avail;
                L1C0 = L3A0;
                L1C1 = L3A1;
                L1C2 = L3A2;
                L1C3 = L3A3;
                L1DxMin = L3RaMin;
                L1DxMax = L3RaMax;
                L1Type = L3LineType;
                L1DLM = L3DLType;
                L1Width = L3Wid;
                L1Reliable = L3Confidence;
            elseif L3SideType==2
                L2Conf = L3Avail;
                L2C0 = L3A0;
                L2C1 = L3A1;
                L2C2 = L3A2;
                L2C3 = L3A3;
                L2DxMin = L3RaMin;
                L2DxMax = L3RaMax;
                L2Type = L3LineType;
                L2DLM = L3DLType;
                L2Width = L3Wid;
                L2Reliable = L3Confidence;
            elseif L3SideType==3
                L3Conf = L3Avail;
                L3C0 = L3A0;
                L3C1 = L3A1;
                L3C2 = L3A2;
                L3C3 = L3A3;
                L3DxMin = L3RaMin;
                L3DxMax = L3RaMax;
                L3Type = L3LineType;
                L3DLM = L3DLType;
                L3Width = L3Wid;
                L3Reliable = L3Confidence;
            elseif L3SideType==4
                L4Conf = L3Avail;
                L4C0 = L3A0;
                L4C1 = L3A1;
                L4C2 = L3A2;
                L4C3 = L3A3;
                L4DxMin = L3RaMin;
                L4DxMax = L3RaMax;
                L4Type = L3LineType;
                L4DLM = L3DLType;
                L4Width = L3Wid;
                L4Reliable = L3Confidence;
            end
            if LA_Count >= 4
                if L4SideType==1
                    L1Conf = L4Avail;
                    L1C0 = L4A0;
                    L1C1 = L4A1;
                    L1C2 = L4A2;
                    L1C3 = L4A3;
                    L1DxMin = L4RaMin;
                    L1DxMax = L4RaMax;
                    L1Type = L4LineType;
                    L1DLM = L4DLType;
                    L1Width = L4Wid;
                    L1Reliable = L4Confidence;
                elseif L4SideType==2
                    L2Conf = L4Avail;
                    L2C0 = L4A0;
                    L2C1 = L4A1;
                    L2C2 = L4A2;
                    L2C3 = L4A3;
                    L2DxMin = L4RaMin;
                    L2DxMax = L4RaMax;
                    L2Type = L4LineType;
                    L2DLM = L4DLType;
                    L2Width = L4Wid;
                    L2Reliable = L4Confidence;
                elseif L4SideType==3
                    L3Conf = L4Avail;
                    L3C0 = L4A0;
                    L3C1 = L4A1;
                    L3C2 = L4A2;
                    L3C3 = L4A3;
                    L3DxMin = L4RaMin;
                    L3DxMax = L4RaMax;
                    L3Type = L4LineType;
                    L3DLM = L4DLType;
                    L3Width = L4Wid;
                    L3Reliable = L4Confidence;
                elseif L4SideType==4
                    L4Conf = L4Avail;
                    L4C0 = L4A0;
                    L4C1 = L4A1;
                    L4C2 = L4A2;
                    L4C3 = L4A3;
                    L4DxMin = L4RaMin;
                    L4DxMax = L4RaMax;
                    L4Type = L4LineType;
                    L4DLM = L4DLType;
                    L4Width = L4Wid;
                    L4Reliable = L4Confidence;
                end
            end
        end
    end
end

== matlab function Noa_Nofusion_angle/Chassis1/Subsystem/CheckSum8Bclc4 ==
  data: Data input; MsgByte output; DataID input
function MsgByte  = CheckSum8B(Data,DataID)
CRC_8_H1D_Tbl =[ 0x00, 0x1d, 0x3a, 0x27, 0x74, 0x69, 0x4e, 0x53, 0xe8, 0xf5, 0xd2, 0xcf, 0x9c, 0x81, 0xa6, 0xbb,...
    0xcd, 0xd0, 0xf7, 0xea, 0xb9, 0xa4, 0x83, 0x9e, 0x25, 0x38, 0x1f, 0x02, 0x51, 0x4c, 0x6b, 0x76, 0x87, 0x9a, 0xbd, 0xa0, 0xf3, 0xee, 0xc9, 0xd4,...
    0x6f, 0x72, 0x55, 0x48, 0x1b, 0x06, 0x21, 0x3c, 0x4a, 0x57, 0x70, 0x6d, 0x3e, 0x23, 0x04, 0x19, 0xa2, 0xbf, 0x98, 0x85, 0xd6, 0xcb, 0xec, 0xf1,...
    0x13, 0x0e, 0x29, 0x34, 0x67, 0x7a, 0x5d, 0x40, 0xfb, 0xe6, 0xc1, 0xdc, 0x8f, 0x92, 0xb5, 0xa8, 0xde, 0xc3, 0xe4, 0xf9, 0xaa, 0xb7, 0x90, 0x8d,...
    0x36, 0x2b, 0x0c, 0x11, 0x42, 0x5f, 0x78, 0x65, 0x94, 0x89, 0xae, 0xb3, 0xe0, 0xfd, 0xda, 0xc7, 0x7c, 0x61, 0x46, 0x5b, 0x08, 0x15, 0x32, 0x2f,...
    0x59, 0x44, 0x63, 0x7e, 0x2d, 0x30, 0x17, 0x0a, 0xb1, 0xac, 0x8b, 0x96, 0xc5, 0xd8, 0xff, 0xe2, 0x26, 0x3b, 0x1c, 0x01, 0x52, 0x4f, 0x68, 0x75,...
    0xce, 0xd3, 0xf4, 0xe9, 0xba, 0xa7, 0x80, 0x9d, 0xeb, 0xf6, 0xd1, 0xcc, 0x9f, 0x82, 0xa5, 0xb8, 0x03, 0x1e, 0x39, 0x24, 0x77, 0x6a, 0x4d, 0x50,...
    0xa1, 0xbc, 0x9b, 0x86, 0xd5, 0xc8, 0xef, 0xf2, 0x49, 0x54, 0x73, 0x6e, 0x3d, 0x20, 0x07, 0x1a, 0x6c, 0x71, 0x56, 0x4b, 0x18, 0x05, 0x22, 0x3f,...
    0x84, 0x99, 0xbe, 0xa3, 0xf0, 0xed, 0xca, 0xd7, 0x35, 0x28, 0x0f, 0x12, 0x41, 0x5c, 0x7b, 0x66, 0xdd, 0xc0, 0xe7, 0xfa, 0xa9, 0xb4, 0x93, 0x8e,...
    0xf8, 0xe5, 0xc2, 0xdf, 0x8c, 0x91, 0xb6, 0xab, 0x10, 0x0d, 0x2a, 0x37, 0x64, 0x79, 0x5e, 0x43, 0xb2, 0xaf, 0x88, 0x95, 0xc6, 0xdb, 0xfc, 0xe1,...
    0x5a, 0x47, 0x60, 0x7d, 0x2e, 0x33, 0x14, 0x09, 0x7f, 0x62, 0x45, 0x58, 0x0b, 0x16, 0x31, 0x2c, 0x97, 0x8a, 0xad, 0xb0, 0xe3, 0xfe, 0xd9, 0xc4];

CRC_temp=uint8(zeros(1));

for t_index = 1:2
    CRC_temp = bitxor(DataID(t_index),CRC_temp);
    CRC_temp = CRC_8_H1D_Tbl(CRC_temp+1);
end

for t_index = 10:16
    CRC_temp = bitxor(Data(t_index),CRC_temp);
    CRC_temp = CRC_8_H1D_Tbl(CRC_temp+1);
end
Data(9)=CRC_temp;
CRC_temp=uint8(zeros(1));
for t_index = 3:4
    CRC_temp = bitxor(DataID(t_index),CRC_temp);
    CRC_temp = CRC_8_H1D_Tbl(CRC_temp+1);
end

for t_index = 18:24
    CRC_temp = bitxor(Data(t_index),CRC_temp);
    CRC_temp = CRC_8_H1D_Tbl(CRC_temp+1);
end
Data(17)=CRC_temp;
MsgByte=Data;
end

== matlab function Noa_Nofusion_angle/TOS/Subsystem1/ACCOSM/ObjMatrixTransit/Subsystem/MATLAB Function1 ==
  data: P output uint8; Count input uint8 size=1; ID input uint8 size=20; BrakeLight_b input uint8 size=20; Class input uint8 size=20; LatDis input single size=20; LatVel input single size=20; LongAccel input single size=20; LongDis input single size=20; LongVel input single size=20; Width input single size=20; Age input uint16 size=20; MotionSts input uint8 size=20; ObjValid output boolean size=20; ObjBrakeLightIndic output uint8 size=20; ObjClassification output uint8 size=20; ObjLatPos output single size=20; ObjLatVel output single size=20; ObjLongAccel output single size=20; ObjLongVel output single size=20; ObjWidth output single size=20; ObjCnt output uint8 size=20; ObjMoveSts output uint8 size=20; ObjLongPos output single size=20; ObjIDK1 input uint8 size=20; ObjID output uint8 size=20
function [P,ObjValid,ObjBrakeLightIndic,ObjClassification,...
    ObjLatPos,ObjLatVel,ObjLongAccel,ObjLongVel,...
    ObjWidth,ObjCnt,ObjMoveSts,ObjLongPos,ObjID] =...
    DataT(Count,ID,BrakeLight_b,Class,LatDis,LatVel,LongAccel,LongDis,LongVel,Width,Age,MotionSts,ObjIDK1)

ObjValid = false(20,1);
ObjID = uint8(zeros(20,1));
ObjBrakeLightIndic = uint8(zeros(20,1));
ObjClassification = uint8(zeros(20,1));
ObjLatPos = single(zeros(20,1));
ObjLatVel = single(zeros(20,1));
ObjLongAccel = single(zeros(20,1));
ObjLongPos = single(zeros(20,1));
ObjLongVel = single(zeros(20,1));
ObjWidth = single(zeros(20,1));
ObjCnt = uint8(zeros(20,1));
ObjMoveSts = uint8(zeros(20,1));

T = uint8(zeros(20,1));
P = uint8(zeros(20,1));
Index01 = uint8(zeros(20,1));
Index02 = uint8(zeros(20,1));
M = uint8(0);
N = uint8(0);
w = uint8(0);

for i=uint8(1):Count
    for j=uint8(1):uint8(20)
        if ID(i)==ObjIDK1(j)
            T(j) = i;
            P(i) = j;
        end
    end
end

for j=uint8(1):uint8(20)
    if T(j)==uint8(0)
        if ObjIDK1(j)==uint8(0)
            N = N + uint8(1);
            Index01(N) = j;
        else
            M = M + uint8(1);
            Index02(M) = j;
        end
        ObjValid(j) = false;
    else
        ObjValid(j) = true;
    end
end

for i=uint8(1):Count
    if P(i)==uint8(0)
        w = w + uint8(1);
        if w<=N
            P(i) = Index01(w);
        else
            P(i) = Index02(w - N);
        end
        ObjValid(Index01(w)) = true;
    end
    ObjID(P(i)) = ID(i);
    if BrakeLight_b(i)==uint8(1)
        ObjBrakeLightIndic(P(i)) = uint8(2);
    end
    if Class(i)==uint8(1)||Class(i)==uint8(2)||...
            Class(i)==uint8(3)||Class(i)==uint8(6)
        ObjClassification(P(i)) = uint8(1);
    end
    ObjLatPos(P(i)) = -LatDis(i) - single(0.1);
    ObjLatVel(P(i)) = -LatVel(i);
    ObjLongAccel(P(i)) = LongAccel(i);
    ObjLongPos(P(i)) = LongDis(i);
    ObjLongVel(P(i)) = LongVel(i);
    ObjWidth(P(i)) = Width(i);
    if Age(i)<=255
        ObjCnt(P(i)) = uint8(Age(i)/2) - uint8(1);
    else
        ObjCnt(P(i)) = uint8(127);
    end
    if MotionSts(i)==uint8(1)||MotionSts(i)==uint8(3)
        ObjMoveSts(P(i)) = uint8(1);
    elseif MotionSts(i)==uint8(2)||MotionSts(i)==uint8(5)
        if LongVel(i)>-2.5
            ObjMoveSts(P(i)) = uint8(2);
        else
            ObjMoveSts(P(i)) = uint8(4);
        end
    elseif MotionSts(i)==uint8(4)
        ObjMoveSts(P(i)) = uint8(3);
    end
end
end

== stateflow chart Noa_Nofusion_angle/TOS/Subsystem1/ACCOSM/ObjMatrixTransit/Subsystem/Obj ==
  (default) -> (junction 5)
  (junction 5) -> (junction 36) : {i=1;}
  (junction 36) -> (junction 38) [order 1] : [i<21]
  (junction 40) -> (junction 36) : {i=i+1;}
  (junction 36) -> (junction 42) [order 2]
  (junction 38) -> (junction 40) : {id(i) = IFV410_Obj(i).OBJ_ID;
      | confidence(i) = IFV410_Obj(i).OBJ_Existence_Probability;
      | classification(i) = IFV410_Obj(i).OBJ_Object_Class;
      | width(i) = IFV410_Obj(i).OBJ_Width;
      | LongDis(i) = IFV410_Obj(i).OBJ_Long_Distance;
      | LatDis(i) = IFV410_Obj(i).OBJ_Lat_Distance;
      | AbsLongAcc(i) = IFV410_Obj(i).OBJ_Abs_Long_Acc;
      | AbsLongVel(i) = IFV410_Obj(i).OBJ_Abs_Long_Velocity;
      | AbsLatVel(i) = IFV410_Obj(i).OBJ_Abs_Lat_Velocity;
      | BrakeLight(i) = IFV410_Obj(i).OBJ_Brake_Light;
      | Age(i) = IFV410_Obj(i).OBJ_Object_Age;
      | motionSts(i) = IFV410_Obj(i).OBJ_Motion_Status;
      | motionCategory(i) = IFV410_Obj(i).OBJ_Motion_Category;
      | motionOrientation(i) = IFV410_Obj(i).OBJ_Motion_Orientation;}
  data: i local uint8; id output uint8 size=20 =uint8(zeros(20,1)); classification output uint8 size=20 =uint8(zeros(20,1)); AbsLongAcc output single size=20 =single(zeros(20,1)); width output single size=20 =single(zeros(20,1)); AbsLongVel output single size=20 =single(zeros(20,1)); LongDis output single size=20 =single(zeros(20,1)); AbsLatVel output single size=20 =single(zeros(20,1)); LatDis output single size=20 =single(zeros(20,1)); BrakeLight output uint8 size=20 =uint8(zeros(20,1)); Age output uint16 size=20 =uint16(zeros(20,1)); confidence output single size=20 =single(zeros(20,1)); IFV410_Obj input Bus: SPI_EQ4_OBJ_ELEM_BUS size=20; motionSts output uint8 size=20 =uint8(zeros(20,1)); motionCategory output uint8 size=20 =uint8(zeros(20,1)); motionOrientation output uint8 size=20 =uint8(zeros(20,1))
